simulink model "Repetitive_Controller"  (R2021b)
settings: Solver=FixedStepDiscrete  StartTime=0.0  StopTime=tspan(2)  FixedStep=0.1  RelTol=1e-3  EnableMultiTasking=on
undefined symbols (not defined in the file): K1, K2, Tmax, x_0
libraries: simulink x1
(part 1 of 2)
settings Model: Creator=domin  LastModifiedBy=domin
settings SolverCC: AlgebraicLoopSolver=TrustRegion  AutoInsertRateTranBlk=on
settings DataIOCC: LimitDataPoints=on
settings OptimizationCC: LifeSpan=inf
settings DebuggingCC: AllowSymbolicDim=off  SFUnexpectedBacktrackingDiag=warning  SFNoUnconditionalDefaultTransitionDiag=warning  SFExecutionAtInitializationDiag=none  ArithmeticOperatorsInVariantConditions=warning
settings SFSimCC: SimUseLocalCustomCode=off  CustomCodeUndefinedFunction=UseInterfaceOnly
settings RTWCC: RTWUseLocalCustomCode=off
settings CodeAppCC: StateflowObjectComments=on
settings GRTTargetCC: TargetLangStandard=C89/C90 (ANSI)
settings ConfigComp: CovMetricSettings=dw  CovSaveCumulativeToWorkspaceVar=on  CovSaveSingleToWorkspaceVar=on  CovExternalEMLEnable=off  CovSFcnEnable=off

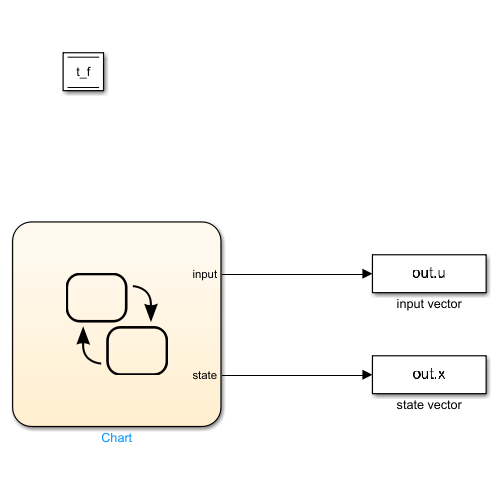
[thumbnail: Simulink's stored preview of the top-level diagram]
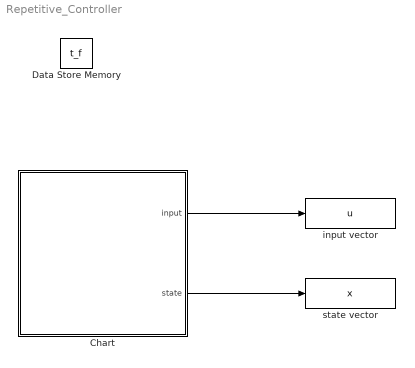
== system Repetitive_Controller ==
  Chart : Stateflow chart  TreatAsAtomicUnit=on
  Data Store Memory : DataStoreMemory  DataStoreName=t_f  ReadBeforeWriteMsg=warning  WriteAfterWriteMsg=warning  WriteAfterReadMsg=warning  ShowAdditionalParam=off
  input vector : ToWorkspace  VariableName=u  SampleTime=-1
  state vector : ToWorkspace  VariableName=x  SampleTime=-1
  wires:
  Chart/2(state) -> state vector/1
  Chart/1(input) -> input vector/1

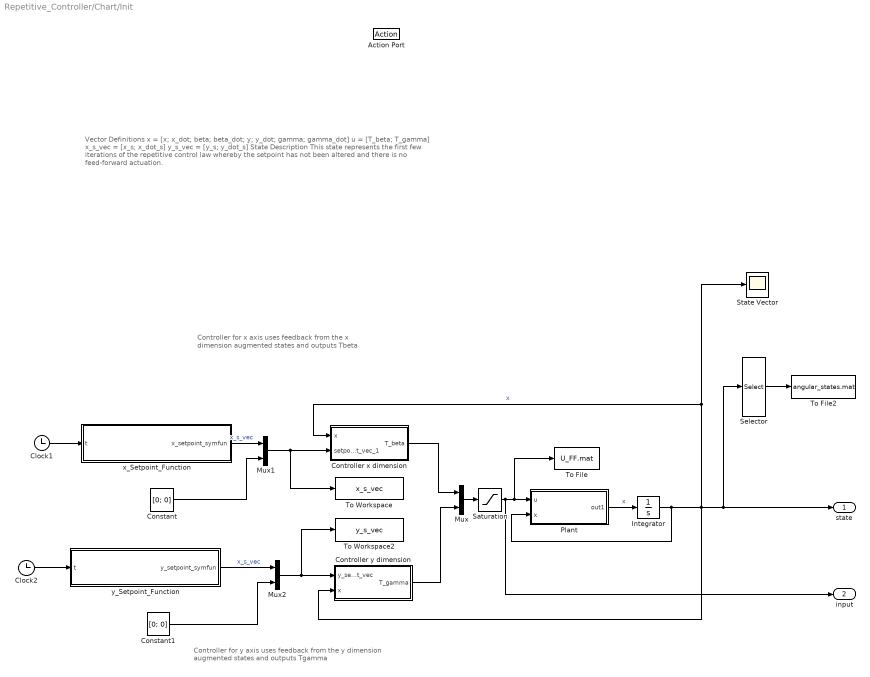
== system Repetitive_Controller/Chart/Init ==
  note: Controller for y axis uses feedback from the
      | y dimension augmented states and outputs Tgamma
  note: Vector Definitions
      |
      | x = [x; x_dot; beta; beta_dot; y; y_dot; gamma; gamma_dot]
      | u = [T_beta; T_gamma]
      | x_s_vec = [x_s; x_dot_s]
      | y_s_vec = [y_s; y_dot_s]
      |
      | State Description
      | This state represents the first few iterations of the repetitive control law whereby the setpoint has not been altered and there is no feed-forward actuation.
  note: Controller for x axis uses feedback from the
      | x dimension augmented states and outputs Tbeta
  Action Port : ActionPort
      settings: CopyFcn=Stateflow.SLINSF.SimulinkMan.removeBlockPreDeleteFcn  PreDeleteFcn=Stateflow.SLINSF.SimulinkMan.unsafePredeleteFcn
  Clock1 : Clock
  Clock2 : Clock
  Constant : Constant  Value=[0; 0]
  Constant1 : Constant  Value=[0; 0]
  Controller x dimension : Subsystem
  Controller y dimension : Subsystem
  Integrator : Integrator  InitialCondition=x_0  ContinuousStateAttributes='x'
  Mux : Mux  Inputs=2
  Mux1 : Mux  Inputs=2
  Mux2 : Mux  Inputs=2
  Plant : Subsystem
  Saturation : Saturate  UpperLimit=Tmax  LowerLimit=-Tmax
  Selector : Selector  InputPortWidth=8  IndexOptions=Index vector (dialog)  Indices=[3 4 7 8]  OutputSizes=1
  State Vector : Scope
  To File : ToFile  Filename=U_FF.mat
  To File2 : ToFile  Filename=angular_states.mat
  To Workspace : ToWorkspace  VariableName=x_s_vec  SampleTime=-1
  To Workspace2 : ToWorkspace  VariableName=y_s_vec  SampleTime=-1
  x_Setpoint_Function : MATLAB Function  TreatAsAtomicUnit=on
  y_Setpoint_Function : MATLAB Function  TreatAsAtomicUnit=on
  state : Outport
  input : Outport  Port=2
  wires:
  Saturation/1 -> input/1, To File/1, Plant/1(u)
  Clock2/1 -> y_Setpoint_Function/1(t)
  Mux/1 -> Saturation/1
  Clock1/1 -> x_Setpoint_Function/1(t)
  Plant/1(out1) -> Integrator/1  "x"
  Controller x dimension/1(T_beta) -> Mux/1
  x_Setpoint_Function/1(x_setpoint_symfun) -> Mux1/1  "x_s_vec"
  Controller y dimension/1(T_gamma) -> Mux/2
  Mux1/1 -> To Workspace/1, Controller x dimension/2(setpoint_vec_1)
  Constant/1 -> Mux1/2
  Mux2/1 -> To Workspace2/1, Controller y dimension/1(y_setpoint_vec)
  y_Setpoint_Function/1(y_setpoint_symfun) -> Mux2/1  "x_s_vec"
  Constant1/1 -> Mux2/2
  Selector/1 -> To File2/1
  Integrator/1 -> Plant/2(x), state/1, Selector/1, Controller x dimension/1(x), State Vector/1, Controller y dimension/2(x)  "x"

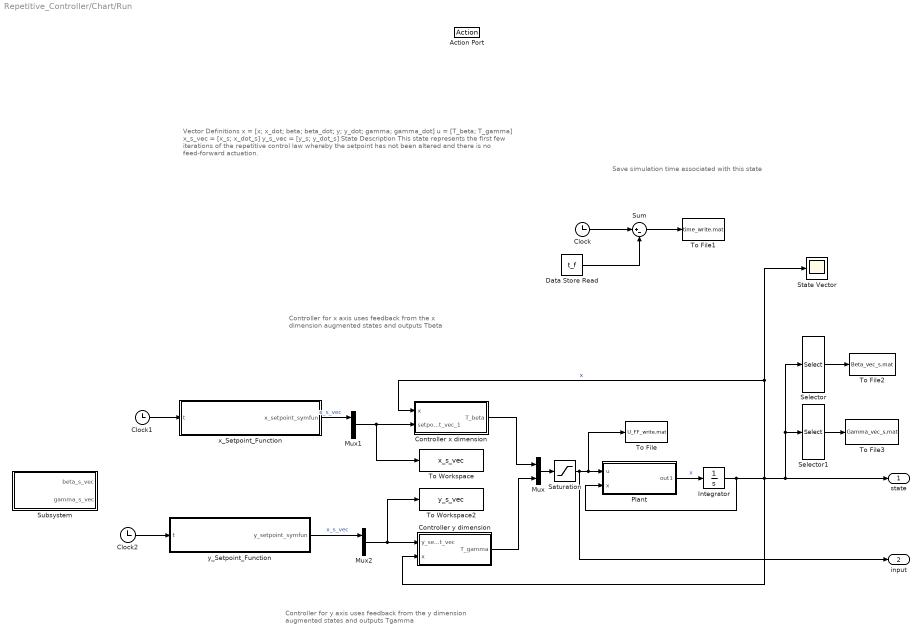
== system Repetitive_Controller/Chart/Run ==
  note: Save simulation time associated with this state
  note: Controller for y axis uses feedback from the
      | y dimension augmented states and outputs Tgamma
  note: Vector Definitions
      |
      | x = [x; x_dot; beta; beta_dot; y; y_dot; gamma; gamma_dot]
      | u = [T_beta; T_gamma]
      | x_s_vec = [x_s; x_dot_s]
      | y_s_vec = [y_s; y_dot_s]
      |
      | State Description
      | This state represents the first few iterations of the repetitive control law whereby the setpoint has not been altered and there is no feed-forward actuation.
  note: Controller for x axis uses feedback from the
      | x dimension augmented states and outputs Tbeta
  Action Port : ActionPort
      settings: CopyFcn=Stateflow.SLINSF.SimulinkMan.removeBlockPreDeleteFcn  PreDeleteFcn=Stateflow.SLINSF.SimulinkMan.unsafePredeleteFcn
  Clock : Clock
  Clock1 : Clock
  Clock2 : Clock
  Controller x dimension : Subsystem
  Controller y dimension : Subsystem
  Data Store Read : DataStoreRead  DataStoreName=t_f  IndexOptions=Index vector (dialog)  Indices=1  OutputSizes=1
  Integrator : Integrator  ContinuousStateAttributes='x'
  Mux : Mux  Inputs=2
  Mux1 : Mux  Inputs=2
  Mux2 : Mux  Inputs=2
  Plant : Subsystem
  Saturation : Saturate  UpperLimit=Tmax  LowerLimit=-Tmax
  Selector : Selector  InputPortWidth=8  IndexOptions=Index vector (dialog)  Indices=[3 4]  OutputSizes=1
  Selector1 : Selector  InputPortWidth=8  IndexOptions=Index vector (dialog)  Indices=[7 8]  OutputSizes=1
  State Vector : Scope
  Subsystem : Subsystem
  Sum : Sum  Inputs=|+-
  To File : ToFile  Filename=U_FF_write.mat
  To File1 : ToFile  Filename=time_write.mat
  To File2 : ToFile  Filename=Beta_vec_s.mat
  To File3 : ToFile  Filename=Gamma_vec_s.mat
  To Workspace : ToWorkspace  VariableName=x_s_vec  SampleTime=-1
  To Workspace2 : ToWorkspace  VariableName=y_s_vec  SampleTime=-1
  x_Setpoint_Function : MATLAB Function  TreatAsAtomicUnit=on
  y_Setpoint_Function : MATLAB Function  TreatAsAtomicUnit=on
  " state" : Outport
  input : Outport  Port=2
  wires:
  Saturation/1 -> input/1, To File/1, Plant/1(u)
  Clock2/1 -> y_Setpoint_Function/1(t)
  Mux/1 -> Saturation/1
  Clock1/1 -> x_Setpoint_Function/1(t)
  Plant/1(out1) -> Integrator/1  "x"
  Controller x dimension/1(T_beta) -> Mux/1
  x_Setpoint_Function/1(x_setpoint_symfun) -> Mux1/1  "x_s_vec"
  Controller y dimension/1(T_gamma) -> Mux/2
  Mux1/1 -> To Workspace/1, Controller x dimension/2(setpoint_vec_1)
  ? -> Mux1/2
  Mux2/1 -> To Workspace2/1, Controller y dimension/1(y_setpoint_vec)
  y_Setpoint_Function/1(y_setpoint_symfun) -> Mux2/1  "x_s_vec"
  ? -> Mux2/2
  Clock/1 -> Sum/1
  Sum/1 -> To File1/1
  Data Store Read/1 -> Sum/2
  Selector/1 -> To File2/1
  Selector1/1 -> To File3/1
  Integrator/1 -> Plant/2(x), " state"/1, Selector1/1, Selector/1, Controller x dimension/1(x), State Vector/1, Controller y dimension/2(x)  "x"

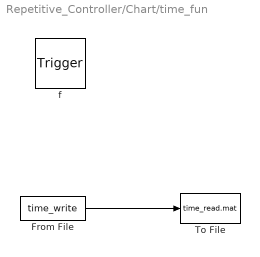
== system Repetitive_Controller/Chart/time_fun ==
  f : TriggerPort  TriggerType=function-call  VariantControl=(inherit)
      settings: CopyFcn=Stateflow.SLINSF.SimulinkMan.removeBlockPreDeleteFcn  PreDeleteFcn=Stateflow.SLINSF.SimulinkMan.unsafePredeleteFcn
  From File : FromFile  FileName=time_write  SampleTime=0
  To File : ToFile  Filename=time_read.mat  SaveFormat=Timeseries
  wires:
  From File/1 -> To File/1

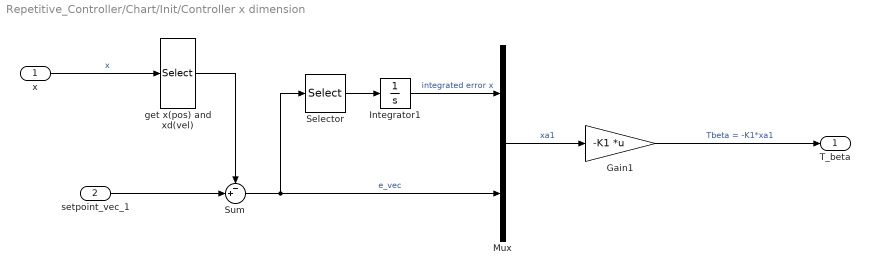
== system Repetitive_Controller/Chart/Init/Controller x dimension ==
  x : Inport
  setpoint_vec_1 : Inport  Port=2
  Gain1 : Gain  Gain=-K1  Multiplication=Matrix(K*u)
  Integrator1 : Integrator
  Mux : Mux  Inputs=2
  Selector : Selector  InputPortWidth=4  IndexOptions=Index vector (dialog)  Indices=[1 ]  OutputSizes=1
  Sum : Sum  Inputs=-+|
  get x(pos) and xd(vel) : Selector  InputPortWidth=8  IndexOptions=Index vector (dialog)  Indices=[1:4]  OutputSizes=1
  T_beta : Outport
  wires:
  Gain1/1 -> T_beta/1  "Tbeta = -K1*xa1"
  get x(pos) and xd(vel)/1 -> Sum/1
  Mux/1 -> Gain1/1  "xa1"
  Sum/1 -> Selector/1, Mux/2  "e_vec"
  setpoint_vec_1/1 -> Sum/2
  x/1 -> get x(pos) and xd(vel)/1  "x"
  Selector/1 -> Integrator1/1
  Integrator1/1 -> Mux/1  "integrated error x"

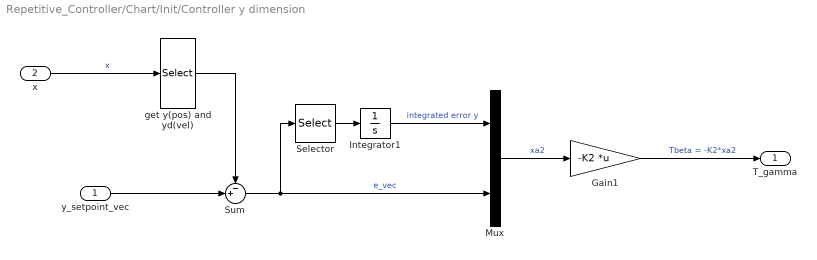
== system Repetitive_Controller/Chart/Init/Controller y dimension ==
  y_setpoint_vec : Inport
  x : Inport  Port=2
  Gain1 : Gain  Gain=-K2  Multiplication=Matrix(K*u)
  Integrator1 : Integrator
  Mux : Mux  Inputs=2
  Selector : Selector  InputPortWidth=4  IndexOptions=Index vector (dialog)  Indices=[1 ]  OutputSizes=1
  Sum : Sum  Inputs=-+|
  get y(pos) and yd(vel) : Selector  InputPortWidth=8  IndexOptions=Index vector (dialog)  Indices=[5:8]  OutputSizes=1
  T_gamma : Outport
  wires:
  Integrator1/1 -> Mux/1  "integrated error y"
  x/1 -> get y(pos) and yd(vel)/1  "x"
  Gain1/1 -> T_gamma/1  "Tbeta = -K2*xa2"
  get y(pos) and yd(vel)/1 -> Sum/1
  Mux/1 -> Gain1/1  "xa2"
  Selector/1 -> Integrator1/1
  Sum/1 -> Selector/1, Mux/2  "e_vec"
  y_setpoint_vec/1 -> Sum/2

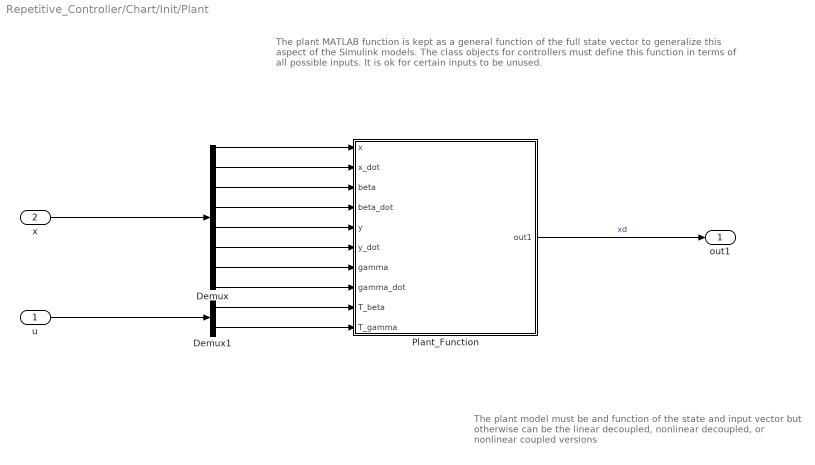
== system Repetitive_Controller/Chart/Init/Plant ==
  note: The plant MATLAB function is kept as a general function of the full state vector
      | to generalize this aspect of the Simulink models. The class objects for controllers must define this function in terms of all possible inputs. It is ok for certain inputs to be unused.
  note: The plant model must be and function of the state and input vector
      |  but otherwise can be the linear decoupled, nonlinear decoupled,
      | or nonlinear coupled versions
  u : Inport
  x : Inport  Port=2
  Demux : Demux  Outputs=8
  Demux1 : Demux  Outputs=2
  Plant_Function : MATLAB Function  TreatAsAtomicUnit=on
  out1 : Outport
  wires:
  Demux1/1 -> Plant_Function/9(T_beta)
  Demux1/2 -> Plant_Function/10(T_gamma)
  Demux/5 -> Plant_Function/5(y)
  Demux/8 -> Plant_Function/8(gamma_dot)
  Demux/7 -> Plant_Function/7(gamma)
  Demux/1 -> Plant_Function/1(x)
  Demux/3 -> Plant_Function/3(beta)
  Demux/4 -> Plant_Function/4(beta_dot)
  Demux/2 -> Plant_Function/2(x_dot)
  Demux/6 -> Plant_Function/6(y_dot)
  x/1 -> Demux/1
  Plant_Function/1(out1) -> out1/1  "xd"
  u/1 -> Demux1/1

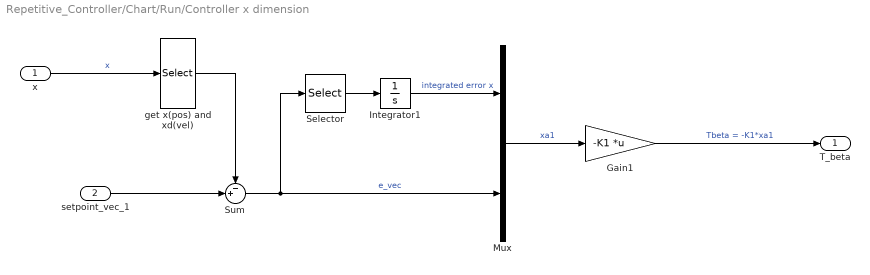
== system Repetitive_Controller/Chart/Run/Controller x dimension ==
  x : Inport
  setpoint_vec_1 : Inport  Port=2
  Gain1 : Gain  Gain=-K1  Multiplication=Matrix(K*u)
  Integrator1 : Integrator
  Mux : Mux  Inputs=2
  Selector : Selector  InputPortWidth=4  IndexOptions=Index vector (dialog)  Indices=[1 ]  OutputSizes=1
  Sum : Sum  Inputs=-+|
  get x(pos) and xd(vel) : Selector  InputPortWidth=8  IndexOptions=Index vector (dialog)  Indices=[1:4]  OutputSizes=1
  T_beta : Outport
  wires:
  Gain1/1 -> T_beta/1  "Tbeta = -K1*xa1"
  get x(pos) and xd(vel)/1 -> Sum/1
  Mux/1 -> Gain1/1  "xa1"
  Sum/1 -> Selector/1, Mux/2  "e_vec"
  setpoint_vec_1/1 -> Sum/2
  x/1 -> get x(pos) and xd(vel)/1  "x"
  Selector/1 -> Integrator1/1
  Integrator1/1 -> Mux/1  "integrated error x"

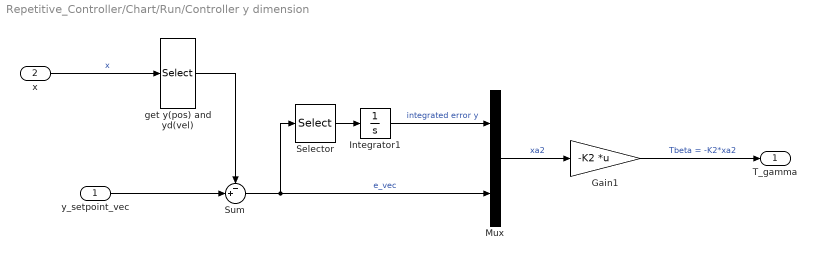
== system Repetitive_Controller/Chart/Run/Controller y dimension ==
  y_setpoint_vec : Inport
  x : Inport  Port=2
  Gain1 : Gain  Gain=-K2  Multiplication=Matrix(K*u)
  Integrator1 : Integrator
  Mux : Mux  Inputs=2
  Selector : Selector  InputPortWidth=4  IndexOptions=Index vector (dialog)  Indices=[1 ]  OutputSizes=1
  Sum : Sum  Inputs=-+|
  get y(pos) and yd(vel) : Selector  InputPortWidth=8  IndexOptions=Index vector (dialog)  Indices=[5:8]  OutputSizes=1
  T_gamma : Outport
  wires:
  Integrator1/1 -> Mux/1  "integrated error y"
  x/1 -> get y(pos) and yd(vel)/1  "x"
  Gain1/1 -> T_gamma/1  "Tbeta = -K2*xa2"
  get y(pos) and yd(vel)/1 -> Sum/1
  Mux/1 -> Gain1/1  "xa2"
  Selector/1 -> Integrator1/1
  Sum/1 -> Selector/1, Mux/2  "e_vec"
  y_setpoint_vec/1 -> Sum/2

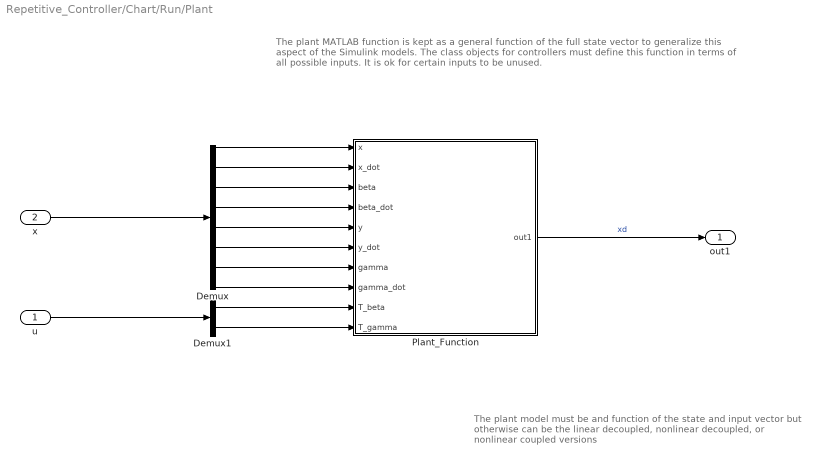
== system Repetitive_Controller/Chart/Run/Plant ==
  note: The plant MATLAB function is kept as a general function of the full state vector
      | to generalize this aspect of the Simulink models. The class objects for controllers must define this function in terms of all possible inputs. It is ok for certain inputs to be unused.
  note: The plant model must be and function of the state and input vector
      |  but otherwise can be the linear decoupled, nonlinear decoupled,
      | or nonlinear coupled versions
  u : Inport
  x : Inport  Port=2
  Demux : Demux  Outputs=8
  Demux1 : Demux  Outputs=2
  Plant_Function : MATLAB Function  TreatAsAtomicUnit=on
  out1 : Outport
  wires:
  Demux1/1 -> Plant_Function/9(T_beta)
  Demux1/2 -> Plant_Function/10(T_gamma)
  Demux/5 -> Plant_Function/5(y)
  Demux/8 -> Plant_Function/8(gamma_dot)
  Demux/7 -> Plant_Function/7(gamma)
  Demux/1 -> Plant_Function/1(x)
  Demux/3 -> Plant_Function/3(beta)
  Demux/4 -> Plant_Function/4(beta_dot)
  Demux/2 -> Plant_Function/2(x_dot)
  Demux/6 -> Plant_Function/6(y_dot)
  x/1 -> Demux/1
  Plant_Function/1(out1) -> out1/1  "xd"
  u/1 -> Demux1/1

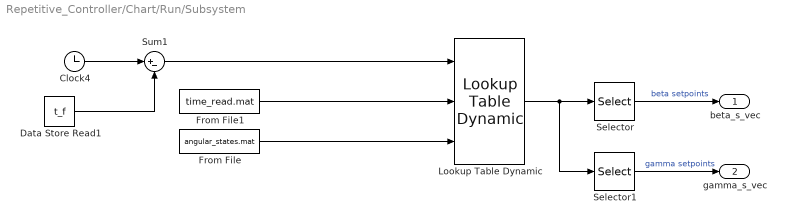
== system Repetitive_Controller/Chart/Run/Subsystem ==
  Clock4 : Clock
  Data Store Read1 : DataStoreRead  DataStoreName=t_f  IndexOptions=Index vector (dialog)  Indices=1  OutputSizes=1
  From File : FromFile  FileName=angular_states.mat  SampleTime=0
  From File1 : FromFile  FileName=time_read.mat  SampleTime=0
  Lookup Table Dynamic : simulink/Lookup Tables/Lookup Table Dynamic  LookUpMeth=Interpolation-Extrapolation  OutDataType=fixdt('double')  OutScaling=2^-10  OutputDataTypeScalingMode=Specify via dialog  OutDataTypeStr=double  DoSatur=off
  Selector : Selector  InputPortWidth=4  IndexOptions=Index vector (dialog)  Indices=[1 2]  OutputSizes=1
  Selector1 : Selector  InputPortWidth=4  IndexOptions=Index vector (dialog)  Indices=[3 4]  OutputSizes=1
  Sum1 : Sum  Inputs=|+-
  beta_s_vec : Outport
  gamma_s_vec : Outport  Port=2
  wires:
  Data Store Read1/1 -> Sum1/2
  From File/1 -> Lookup Table Dynamic/3
  Lookup Table Dynamic/1 -> Selector1/1, Selector/1
  Sum1/1 -> Lookup Table Dynamic/1
  From File1/1 -> Lookup Table Dynamic/2
  Clock4/1 -> Sum1/1
  Selector/1 -> beta_s_vec/1  "beta setpoints"
  Selector1/1 -> gamma_s_vec/1  "gamma setpoints"

== matlab function Repetitive_Controller/Chart/Init/Plant/Plant_Function ==
  data: x input; out1 output size=8; x_dot input; beta input; beta_dot input; y input; y_dot input; gamma input; gamma_dot input; T_beta input; T_gamma input
function out1 = xdot(x,x_dot,beta,beta_dot,y,y_dot,gamma,gamma_dot,T_beta,T_gamma)
%#codegen

%    This function was generated by the Symbolic Math Toolbox version 9.0.
%    10-Dec-2021 15:41:41

t2 = cos(beta);
t3 = cos(gamma);
t4 = sin(beta);
t5 = sin(gamma);
t6 = beta_dot.^2;
t7 = gamma_dot.^2;
t8 = x.^2;
t9 = x.^3;
t10 = y.^2;
t11 = y.^3;
t13 = y.^5;
t12 = t10.^2;
t14 = t3.^2;
t15 = t3.^3;
t17 = t3.^5;
t19 = t5.^2;
t20 = t5.^3;
t22 = t5.^5;
t29 = t3.*t5.*t8.*y.*1.35016875e-1;
t36 = t3.*t5.*y.*2.54260666546875e-1;
t16 = t14.^2;
t18 = t14.^3;
t21 = t19.^2;
t24 = t8.*t19.*1.24425;
t26 = t12.*t14.*t19.*(5.67e+2./1.6e+2);
t27 = t3.*t11.*t20.*7.2646875e-1;
t28 = t5.*t11.*t15.*7.2646875e-1;
t30 = t8.*t10.*t14.*t19.*(5.67e+2./1.6e+2);
t31 = -t29;
t32 = t3.*t8.*t20.*y.*8.61485625e-1;
t33 = t5.*t8.*t15.*y.*8.61485625e-1;
t34 = t10.*t19.*1.240295934375;
t35 = t8.*t14.*4.3410357703125;
t39 = t19.*2.520596373817331e-3;
t42 = t3.*t20.*y.*9.746092345495838e-2;
t43 = t5.*t15.*y.*9.746092345495838e-2;
t44 = t8.*t14.*t19.*2.124794480871038;
t45 = t10.*t14.*t19.*6.487623695046038;
t46 = t14.*2.101722893640155;
t49 = t14.*t19.*8.065797848171603e-1;
t23 = t12.*t21.*(5.67e+2./1.6e+2);
t25 = t8.*t10.*t21.*(5.67e+2./1.6e+2);
t37 = t10.*t21.*4.82620938917175e-1;
t38 = t8.*t21.*4.60827495054675e-1;
t40 = t8.*t16.*1.663966985816362;
t41 = t10.*t16.*6.005002756128863;
t47 = t21.*9.66172446512356e-4;
t48 = t16.*8.056136123706479e-1;
t50 = t23+t24+t25+t26+t27+t28+t30+t31+t32+t33+t34+t35+t36+t37+t38+t39+t40+t41+t42+t43+t44+t45+t46+t47+t48+t49;
t51 = 1.0./t50;
et1 = T_beta.*t3.*(-2.1476413157)-T_beta.*t15.*8.232146510146728e-1+t4.*t14.*7.39780227196038+t4.*t16.*2.835659367822534;
et2 = t4.*t19.*1.76621788765343e-2+t4.*t21.*6.770108357347294e-3-T_beta.*t3.*t19.*8.232146510146728e-1-T_beta.*t10.*t15.*6.1362-T_beta.*t11.*t20.*(3.15e+2./8.0)+beta_dot.*gamma_dot.*t20.*5.337182778960069e-4;
et3 = beta_dot.*gamma_dot.*t22.*2.045801143172306e-4-T_beta.*t5.*y.*1.37810659375e+1-T_beta.*t20.*y.*5.2824348756075-beta_dot.*t20.*y_dot.*4.321022355115425e-3-beta_dot.*t22.*y_dot.*1.65629562259261e-3;
et4 = t4.*t8.*t14.*3.041825779054688e+1+t4.*t8.*t16.*1.165965437918465e+1+t6.*t9.*t14.*3.1007398359375+t4.*t10.*t16.*2.113686022398367e+1+t4.*t8.*t19.*8.7186375+t6.*t9.*t16.*1.188547847011688;
et5 = t4.*t8.*t21.*3.229084090347401+t6.*t9.*t19.*(7.11e+2./8.0e+2)+t4.*t10.*t21.*5.0464042216875e-2+t6.*t9.*t21.*3.29162496467625e-1+t4.*t14.*t19.*2.842429476179882;
et6 = t2.*t3.*x.*(-4.740381294078825)-t2.*t15.*x.*1.817040538452137+t6.*t14.*x.*1.487079216073444+t7.*t14.*x.*6.79406330221695e-2;
et7 = t6.*t16.*x.*6.379545310329106e-1+t7.*t16.*x.*2.604239548484917e-2+t6.*t18.*x.*2.604239548484917e-2+t6.*t19.*x.*1.800425981298094e-3;
et8 = t6.*t21.*x.*6.901231760802543e-4-T_beta.*t5.*t11.*t14.*(3.15e+2./8.0)-T_beta.*t3.*t10.*t19.*6.1362-beta_dot.*gamma_dot.*t5.*t14.*2.313734573036617e-2-beta_dot.*gamma_dot.*t5.*t16.*8.868800321352103e-3;
et9 = beta_dot.*gamma_dot.*t8.*t20.*2.6346105e-1-beta_dot.*gamma_dot.*t11.*t17.*8.497709015898375+beta_dot.*gamma_dot.*t8.*t22.*9.757693045286275e-2+beta_dot.*gamma_dot.*t10.*t20.*4.72552750996875e-2+beta_dot.*gamma_dot.*t10.*t22.*1.963839892085062e-2+beta_dot.*gamma_dot.*t12.*t22.*1.35016875e-1;
et10 = beta_dot.*gamma_dot.*t14.*t20.*(-8.664220207034872e-3)+T_gamma.*t3.*t5.*x.*1.79703e-1-T_beta.*t5.*t14.*y.*5.2824348756075-beta_dot.*gamma_dot.*t15.*y.*2.974158432146889;
et11 = beta_dot.*gamma_dot.*t17.*y.*(-1.140027796021482)-T_gamma.*t14.*x.*y.*6.1362+T_gamma.*t19.*x.*y.*(3.69e+2./3.2e+2)-beta_dot.*t5.*t14.*y_dot.*3.596166371785134-beta_dot.*t5.*t16.*y_dot.*1.378450313419718;
et12 = beta_dot.*t8.*t20.*y_dot.*(-2.133)-beta_dot.*t8.*t22.*y_dot.*7.899899915223e-1-beta_dot.*t10.*t20.*y_dot.*1.240295934375-beta_dot.*t10.*t22.*y_dot.*4.87765081854675e-1-beta_dot.*t12.*t22.*y_dot.*(5.67e+2./1.6e+2)-beta_dot.*t14.*t20.*y_dot.*1.380106609042311;
et13 = beta_dot.*t15.*x.*x_dot.*9.66438592065e-1+beta_dot.*t17.*x.*x_dot.*3.704465929566028e-1-gamma_dot.*t3.*t5.*x_dot.*7.3642620715353e-3-gamma_dot.*t5.*t15.*x_dot.*2.822803038329313e-3;
et14 = gamma_dot.*t3.*t20.*x_dot.*(-2.822803038329313e-3)-gamma_dot.*t11.*t21.*x_dot.*1.35016875e-1-gamma_dot.*t14.*x.*y_dot.*9.66438592065e-1-gamma_dot.*t16.*x.*y_dot.*3.704465929566028e-1-gamma_dot.*t19.*x_dot.*y.*4.72552750996875e-2;
et15 = gamma_dot.*t21.*x_dot.*y.*(-1.811346918845812e-2)-t4.*t5.*t11.*t15.*1.331546137149375e+2-t3.*t4.*t11.*t20.*1.331546137149375e+2+t4.*t8.*t10.*t21.*2.48315625e+1+t4.*t8.*t14.*t19.*1.488873846953206e+1+t6.*t9.*t10.*t21.*(8.1e+1./3.2e+1);
et16 = t4.*t10.*t14.*t19.*2.118732426620054e+1+t6.*t9.*t14.*t19.*1.517710343479313+t2.*t3.*t19.*x.*2.222054701596104+t2.*t3.*t21.*x.*1.258051161599348-t6.*t10.*t14.*x.*1.5029307e-2;
et17 = t7.*t10.*t14.*x.*(-1.5029307e-2)+t6.*t10.*t16.*x.*4.319346296949187-t2.*t11.*t20.*x.*8.691046875e+1+t7.*t10.*t16.*x.*5.5462482e-2-t6.*t10.*t18.*x.*5.5462482e-2+t2.*t11.*t22.*x.*6.207890625e+1+t6.*t10.*t19.*x.*(7.11e+2./8.0e+2)+t2.*t15.*t19.*x.*1.258051161599348;
et18 = t7.*t10.*t19.*x.*(7.11e+2./8.0e+2)+t6.*t10.*t21.*x.*3.34306639405125e-1+t7.*t10.*t21.*x.*3.65641605842625e-1+t6.*t12.*t21.*x.*(8.1e+1./3.2e+1)+t6.*t14.*t19.*x.*5.759809778668214e-1+t7.*t12.*t21.*x.*(8.1e+1./3.2e+1);
et19 = t7.*t14.*t19.*x.*2.604239548484917e-2+t6.*t14.*t21.*x.*1.954403639426509e-3+t6.*t16.*t19.*x.*2.799679912427568e-2-t3.*t4.*t5.*y.*4.660349235524814e+1;
et20 = t4.*t5.*t15.*y.*(-1.786363365932268e+1)-t3.*t4.*t20.*y.*1.786363365932268e+1-t2.*t5.*x.*y.*3.041825779054688e+1+t2.*t20.*x.*y.*1.425856456363003e+1;
et21 = t2.*t22.*x.*y.*8.072710225868503+beta_dot.*gamma_dot.*t5.*t8.*t14.*9.191833169653125e-1+beta_dot.*gamma_dot.*t5.*t8.*t16.*3.523331237681446e-1+beta_dot.*gamma_dot.*t5.*t10.*t14.*9.4510550199375e-2-beta_dot.*gamma_dot.*t5.*t10.*t16.*2.988064664334938e-2;
et22 = beta_dot.*gamma_dot.*t5.*t12.*t16.*2.7003375e-1-beta_dot.*gamma_dot.*t3.*t11.*t21.*8.535675761148375+beta_dot.*gamma_dot.*t8.*t10.*t22.*7.5036375e-1+beta_dot.*gamma_dot.*t8.*t14.*t20.*4.499100542210074e-1-beta_dot.*gamma_dot.*t10.*t14.*t20.*1.024224772249876e-2-beta_dot.*gamma_dot.*t11.*t15.*t19.*1.703338477704675e+1;
et23 = beta_dot.*gamma_dot.*t12.*t14.*t20.*4.05050625e-1-T_gamma.*t3.*t5.*t10.*x.*(3.15e+2./8.0)-beta_dot.*gamma_dot.*t3.*t19.*y.*2.987446615504921-beta_dot.*gamma_dot.*t8.*t15.*y.*6.201479671875-beta_dot.*gamma_dot.*t3.*t21.*y.*1.145121303557277-beta_dot.*gamma_dot.*t8.*t17.*y.*2.377095694023375;
et24 = beta_dot.*gamma_dot.*t15.*t19.*y.*(-2.285149099578759)-beta_dot.*t5.*t8.*t14.*y_dot.*7.44177560625-beta_dot.*t5.*t8.*t16.*y_dot.*2.85251483282805-beta_dot.*t5.*t10.*t16.*y_dot.*1.027489829387805e+1-beta_dot.*t3.*t11.*t21.*y_dot.*7.2646875e-1-beta_dot.*t8.*t10.*t22.*y_dot.*(2.43e+2./4.0e+1);
et25 = beta_dot.*t8.*t14.*t20.*y_dot.*(-3.64250482435035)-beta_dot.*t10.*t14.*t20.*y_dot.*1.076266337573272e+1-beta_dot.*t11.*t15.*t19.*y_dot.*7.2646875e-1-beta_dot.*t12.*t14.*t20.*y_dot.*(5.67e+2./1.6e+2)+beta_dot.*t3.*t19.*x.*x_dot.*1.385028e-1+beta_dot.*t3.*t21.*x.*x_dot.*5.129668344951468e-2+beta_dot.*t11.*t22.*x.*x_dot.*(8.1e+1./3.2e+1);
et26 = beta_dot.*t15.*t19.*x.*x_dot.*4.217432764061174e-1-gamma_dot.*t5.*t10.*t15.*x_dot.*2.10410298e-2-gamma_dot.*t3.*t10.*t20.*x_dot.*2.10410298e-2-gamma_dot.*t11.*t14.*t19.*x_dot.*1.35016875e-1-beta_dot.*t3.*t19.*y.*y_dot.*2.54260666546875e-1-beta_dot.*t3.*t21.*y.*y_dot.*9.746092345495838e-2;
et27 = beta_dot.*t15.*t19.*y.*y_dot.*(-9.746092345495838e-2)+beta_dot.*t20.*x.*x_dot.*y.*(7.11e+2./8.0e+2)+beta_dot.*t22.*x.*x_dot.*y.*3.29162496467625e-1-gamma_dot.*t10.*t21.*x.*y_dot.*5.1890625e-1-gamma_dot.*t14.*t19.*x.*y_dot.*3.704465929566028e-1-gamma_dot.*t14.*t19.*x_dot.*y.*1.811346918845812e-2;
et28 = t4.*t8.*t10.*t14.*t19.*2.48315625e+1+t6.*t9.*t10.*t14.*t19.*(8.1e+1./3.2e+1)-t3.*t5.*t6.*t11.*x.*9.6440625e-2-t3.*t5.*t7.*t11.*x.*9.6440625e-2-t2.*t3.*t10.*t19.*x.*1.591929901524375e+2+t2.*t3.*t10.*t21.*x.*1.840267096875e+1+t5.*t6.*t11.*t15.*x.*7.117875e-1+t5.*t7.*t11.*t15.*x.*7.5036375e-1-t5.*t6.*t11.*t17.*x.*7.5036375e-1;
et29 = t3.*t6.*t11.*t20.*x.*6.15346875e-1+t3.*t7.*t11.*t20.*x.*7.5036375e-1+t3.*t6.*t11.*t22.*x.*6.15346875e-1+t2.*t10.*t15.*t19.*x.*1.840267096875e+1+t2.*t11.*t14.*t20.*x.*6.207890625e+1+t6.*t10.*t14.*t19.*x.*9.947678913416812+t7.*t10.*t14.*t19.*x.*4.21104087842625e-1;
et30 = t6.*t10.*t14.*t21.*x.*2.19386751580575+t6.*t10.*t16.*t19.*x.*2.13840503380575+t6.*t12.*t14.*t19.*x.*(8.1e+1./3.2e+1)-t6.*t11.*t15.*t20.*x.*1.35016875e-1+t7.*t12.*t14.*t19.*x.*(8.1e+1./3.2e+1)-t6.*t12.*t14.*t21.*x.*(8.1e+1./3.2e+1)-t6.*t12.*t16.*t19.*x.*(8.1e+1./3.2e+1)-t3.*t4.*t5.*t8.*y.*9.4608253125e-1-t3.*t5.*t6.*t9.*y.*9.6440625e-2;
et31 = t4.*t5.*t8.*t15.*y.*6.03655284375+t3.*t4.*t8.*t20.*y.*6.03655284375+t5.*t6.*t9.*t15.*y.*6.15346875e-1+t3.*t6.*t9.*t20.*y.*6.15346875e-1+t3.*t5.*t6.*x.*y.*9.12475249003125e-2+t3.*t5.*t7.*x.*y.*5.744668209328125e-1-t2.*t5.*t14.*x.*y.*3.435757314273251e+1;
et32 = t2.*t5.*t16.*x.*y.*1.36021737105+t5.*t6.*t15.*x.*y.*1.296510410662169+t5.*t7.*t15.*x.*y.*2.240914151443579e-1+t5.*t6.*t17.*x.*y.*4.940577617661313e-1+t3.*t6.*t20.*x.*y.*6.704458926105656e-2;
et33 = t3.*t7.*t20.*x.*y.*2.240914151443579e-1+t3.*t6.*t22.*x.*y.*1.254109111541651e-2+t2.*t14.*t20.*x.*y.*9.432927596918503+t6.*t15.*t20.*x.*y.*5.065988528815479e-1-beta_dot.*t8.*t10.*t14.*t20.*y_dot.*(2.43e+2./4.0e+1)-beta_dot.*t3.*t10.*t19.*x.*x_dot.*9.6440625e-2;
et34 = beta_dot.*t3.*t10.*t21.*x.*x_dot.*1.26927+beta_dot.*t10.*t15.*t19.*x.*x_dot.*1.26927+beta_dot.*t11.*t14.*t20.*x.*x_dot.*(8.1e+1./3.2e+1)+beta_dot.*t3.*t8.*t19.*y.*y_dot.*2.314575e-1-beta_dot.*t3.*t8.*t21.*y.*y_dot.*1.4768325-beta_dot.*t8.*t15.*t19.*y.*y_dot.*1.4768325+beta_dot.*t5.*t14.*x.*x_dot.*y.*6.186450364875+beta_dot.*t5.*t16.*x.*x_dot.*y.*2.513424526023375;
et35 = beta_dot.*t14.*t20.*x.*x_dot.*y.*2.842587022491-gamma_dot.*t10.*t14.*t19.*x.*y_dot.*5.1890625e-1-gamma_dot.*t3.*t5.*x.*y.*y_dot.*6.201479671875-gamma_dot.*t5.*t15.*x.*y.*y_dot.*2.457962044023375-gamma_dot.*t3.*t20.*x.*y.*y_dot.*2.457962044023375+beta_dot.*gamma_dot.*t5.*t8.*t10.*t14.*1.9288125e-1-beta_dot.*gamma_dot.*t5.*t8.*t10.*t16.*1.23069375;
et36 = beta_dot.*gamma_dot.*t3.*t8.*t11.*t21.*(-8.1e+1./1.6e+1)-beta_dot.*gamma_dot.*t8.*t10.*t14.*t20.*4.8033e-1-beta_dot.*gamma_dot.*t8.*t11.*t15.*t19.*(8.1e+1./1.6e+1)-beta_dot.*gamma_dot.*t3.*t8.*t19.*y.*1.806088858875-beta_dot.*gamma_dot.*t3.*t8.*t21.*y.*4.7591156531025e-1-beta_dot.*gamma_dot.*t8.*t15.*t19.*y.*2.853007259333625;
et37 = T_beta.*(-1.92934923125e+1)-T_beta.*t14.*7.3954088258505-T_beta.*t19.*7.3954088258505-t3.*t4.*6.584303391854071e+1-t4.*t15.*2.523836256676404e+1;
et38 = t2.*x.*(-4.258556090676563e+1)-T_beta.*t10.*t14.*(4.41e+2./8.0)-T_beta.*t10.*t19.*(4.41e+2./8.0)+T_gamma.*t5.*x.*1.614375-gamma_dot.*t5.*x_dot.*6.61573851395625e-2-gamma_dot.*t20.*x_dot.*2.535885686384136e-2-t3.*t4.*t19.*2.523836256676404e+1;
et39 = t4.*t10.*t15.*(-1.881254666584125e+2)-t4.*t11.*t20.*3.47641875e+1-t3.*t6.*x.*1.271303332734375e-1+t3.*t7.*x.*6.103496293059375e-1-t2.*t14.*x.*1.632351613085852e+1+t2.*t19.*x.*1.996199038908205e+1;
et40 = t6.*t15.*x.*5.616191675784583e-1+t7.*t15.*x.*2.339537582057806e-1+t2.*t21.*x.*1.13017943162159e+1+t6.*t17.*x.*2.339537582057806e-1-t4.*t5.*y.*1.216730311621875e+1;
et41 = t4.*t20.*y.*(-4.663861751673862)-beta_dot.*gamma_dot.*t3.*t5.*4.20576885660421-beta_dot.*gamma_dot.*t5.*t15.*1.6121176828866;
et42 = beta_dot.*gamma_dot.*t3.*t20.*(-1.6121176828866)+beta_dot.*gamma_dot.*t11.*t16.*7.2646875e-1-beta_dot.*gamma_dot.*t11.*t21.*8.61485625e-1+beta_dot.*gamma_dot.*t14.*y.*2.54260666546875e-1+beta_dot.*gamma_dot.*t16.*y.*9.746092345495838e-2-beta_dot.*gamma_dot.*t19.*y.*3.015159416465625e-1;
et43 = beta_dot.*gamma_dot.*t21.*y.*(-1.155743926434165e-1)-T_gamma.*t3.*x.*y.*(4.41e+2./8.0)+beta_dot.*t3.*t5.*y_dot.*6.0972948133875e-2+beta_dot.*t5.*t15.*y_dot.*2.337160486363782e-2+beta_dot.*t3.*t20.*y_dot.*2.337160486363782e-2+beta_dot.*t11.*t21.*y_dot.*(5.67e+2./1.6e+2);
et44 = beta_dot.*t14.*x.*x_dot.*8.682071540625+beta_dot.*t16.*x.*x_dot.*3.327933971632725+beta_dot.*t19.*x.*x_dot.*1.24425+beta_dot.*t21.*x.*x_dot.*4.60827495054675e-1-gamma_dot.*t5.*t14.*x_dot.*2.535885686384136e-2-gamma_dot.*t10.*t20.*x_dot.*1.89023625e-1+beta_dot.*t19.*y.*y_dot.*1.240295934375;
et45 = beta_dot.*t21.*y.*y_dot.*4.75419138804675e-1-gamma_dot.*t3.*x.*y_dot.*8.682071540625-gamma_dot.*t15.*x.*y_dot.*3.327933971632725-t4.*t5.*t11.*t14.*3.47641875e+1-t3.*t4.*t10.*t19.*1.881254666584125e+2-t3.*t6.*t10.*x.*1.35016875e-1-t3.*t7.*t10.*x.*1.35016875e-1;
et46 = t3.*t6.*t19.*x.*(-1.324536727479187e-3)+t3.*t7.*t19.*x.*2.339537582057806e-1+t3.*t6.*t21.*x.*1.755752756158312e-2-t2.*t10.*t19.*x.*1.2167465625e+2+t6.*t10.*t15.*x.*2.7003375e-1+t7.*t10.*t15.*x.*4.9825125e-1+t2.*t10.*t21.*x.*8.691046875e+1;
et47 = t6.*t10.*t17.*x.*(-4.9825125e-1)+t2.*t14.*t19.*x.*1.13017943162159e+1+t7.*t11.*t20.*x.*(5.67e+2./1.6e+2)+t6.*t15.*t19.*x.*2.515112857673637e-1-t4.*t5.*t14.*y.*4.663861751673862+t5.*t6.*x.*y.*3.954065625e-3+t5.*t7.*x.*y.*1.24425;
et48 = t6.*t20.*x.*y.*(-1.459164375e-2)+t7.*t20.*x.*y.*5.11898248179675e-1+beta_dot.*gamma_dot.*t3.*t5.*t10.*2.48059186875-beta_dot.*gamma_dot.*t5.*t10.*t15.*1.106580466422338e+1+beta_dot.*gamma_dot.*t5.*t12.*t15.*(5.67e+2./8.0e+1)-beta_dot.*gamma_dot.*t3.*t10.*t20.*1.106580466422338e+1+beta_dot.*gamma_dot.*t3.*t12.*t20.*(5.67e+2./8.0e+1);
et49 = beta_dot.*gamma_dot.*t11.*t14.*t19.*(-1.35016875e-1)-beta_dot.*gamma_dot.*t14.*t19.*y.*1.811346918845812e-2+beta_dot.*t5.*t10.*t15.*y_dot.*1.7421075e-1+beta_dot.*t3.*t10.*t20.*y_dot.*1.7421075e-1+beta_dot.*t11.*t14.*t19.*y_dot.*(5.67e+2./1.6e+2)+beta_dot.*t10.*t21.*x.*x_dot.*(5.67e+2./1.6e+2)+beta_dot.*t14.*t19.*x.*x_dot.*3.7887614666874-gamma_dot.*t5.*t10.*t14.*x_dot.*1.89023625e-1;
et50 = beta_dot.*t14.*t19.*y.*y_dot.*4.75419138804675e-1-gamma_dot.*t3.*t19.*x.*y_dot.*3.327933971632725-gamma_dot.*t20.*x.*y.*y_dot.*7.2646875e-1+t5.*t7.*t11.*t14.*x.*(5.67e+2./1.6e+2)+t3.*t6.*t10.*t19.*x.*1.35016875e-1-t5.*t6.*t11.*t16.*x.*(5.67e+2./1.6e+2)+t3.*t7.*t10.*t19.*x.*4.9825125e-1+t3.*t6.*t10.*t21.*x.*8.61485625e-1+t2.*t10.*t14.*t19.*x.*8.691046875e+1;
et51 = t6.*t10.*t15.*t19.*x.*3.63234375e-1-t6.*t11.*t14.*t20.*x.*(5.67e+2./1.6e+2)-t2.*t3.*t5.*x.*y.*2.039084077834125e+2+t2.*t5.*t15.*x.*y.*1.221961190625e+1+t2.*t3.*t20.*x.*y.*1.221961190625e+1+t5.*t6.*t14.*x.*y.*7.4180857539375+t5.*t7.*t14.*x.*y.*5.11898248179675e-1;
et52 = t5.*t6.*t16.*x.*y.*2.93716060232805+t6.*t14.*t20.*x.*y.*2.93716060232805+beta_dot.*t10.*t14.*t19.*x.*x_dot.*(5.67e+2./1.6e+2)-beta_dot.*t3.*t5.*x.*x_dot.*y.*1.35016875e-1+beta_dot.*t5.*t15.*x.*x_dot.*y.*1.22472+beta_dot.*t3.*t20.*x.*x_dot.*y.*1.22472-gamma_dot.*t5.*t14.*x.*y.*y_dot.*7.2646875e-1;
et53 = T_gamma.*t14.*2.970855966714673+T_gamma.*t19.*3.5629477128e-3-t2.*t20.*4.713080655351523e-3-t2.*t22.*7.559910412543251e-3+T_gamma.*t8.*t14.*6.1362+T_gamma.*t8.*t19.*6.00075e-1;
et54 = T_gamma.*t10.*t19.*1.7532+T_beta.*t5.*x.*1.38478628575e+1+T_beta.*t20.*x.*5.0359349556075+beta_dot.*t20.*x_dot.*4.329749032049133e-3+beta_dot.*t22.*x_dot.*1.624091665194202e-3+t2.*t5.*t8.*3.056569529221687e+1;
et55 = t2.*t5.*t14.*(-3.929859463347265)-t2.*t5.*t16.*6.30360217643565-t5.*t6.*t15.*2.260152122742151e-2;
et56 = t5.*t6.*t17.*(-9.792752004982599e-3)-t3.*t6.*t20.*2.710600556380867e-5-t2.*t8.*t20.*1.725481027987207e+1;
et57 = t3.*t6.*t22.*(-1.174444798034242e-5)-t2.*t8.*t22.*1.13017943162159e+1-t2.*t10.*t20.*2.31913956392829+t6.*t11.*t16.*4.289287682949187;
et58 = t2.*t10.*t22.*(-3.770427399426776)+t7.*t11.*t16.*4.289287682949187-t6.*t11.*t18.*4.289287682949187-t2.*t12.*t22.*2.48315625e+1-t2.*t14.*t20.*6.311162086848193;
et59 = t6.*t11.*t19.*8.90219755125e-1+t7.*t11.*t19.*8.90219755125e-1+t6.*t11.*t21.*3.28882818655125e-1+t7.*t11.*t21.*3.84345300655125e-1+t6.*t13.*t21.*(8.1e+1./3.2e+1)-t6.*t15.*t20.*9.804496452962942e-3+t7.*t13.*t21.*(8.1e+1./3.2e+1);
et60 = t2.*t15.*y.*(-6.557421832530962)+t6.*t14.*y.*1.508507113392871+t7.*t14.*y.*1.508507113392871-t6.*t16.*y.*9.599211127015562e-1;
et61 = t7.*t16.*y.*6.425690291983333e-1-t6.*t18.*y.*4.546029721842959e-1+t6.*t19.*y.*1.809152658231802e-3+t7.*t19.*y.*1.809152658231802e-3;
et62 = t6.*t21.*y.*6.579192186818463e-4+t7.*t21.*y.*7.706330695762743e-4+T_beta.*t5.*t14.*x.*5.0359349556075+T_beta.*t10.*t20.*x.*(3.15e+2./8.0)+T_gamma.*t3.*t5.*y.*3.59406e-1+T_beta.*t15.*x.*y.*6.1362;
et63 = beta_dot.*t5.*t14.*x_dot.*3.610230007033025+beta_dot.*t5.*t16.*x_dot.*1.354199613061963+beta_dot.*t8.*t20.*x_dot.*1.24425+beta_dot.*t8.*t22.*x_dot.*4.60827495054675e-1+beta_dot.*t10.*t20.*x_dot.*2.1305156895;
et64 = beta_dot.*t10.*t22.*x_dot.*8.115037575723e-1+beta_dot.*t12.*t22.*x_dot.*(2.43e+2./4.0e+1)+beta_dot.*t14.*t20.*x_dot.*1.355823704727157+beta_dot.*t17.*x_dot.*y.*1.336885185021603-gamma_dot.*t11.*t21.*y_dot.*7.8894e-1+gamma_dot.*t19.*x.*x_dot.*4.74843217383675e-2;
et65 = gamma_dot.*t21.*x.*x_dot.*1.726822096277812e-2-gamma_dot.*t16.*y.*y_dot.*1.336885185021603-gamma_dot.*t21.*y.*y_dot.*1.60332647076e-3+t3.*t5.*t6.*t8.*9.12475249003125e-2-t3.*t5.*t7.*t8.*4.380771414970125e-1;
et66 = t3.*t5.*t6.*t10.*1.82495049800625e-1+t3.*t5.*t7.*t10.*1.82495049800625e-1+t2.*t5.*t8.*t14.*2.998578957015639-t2.*t5.*t8.*t16.*1.301987175023465e+1-t2.*t5.*t10.*t14.*7.932988935e-1;
et67 = t2.*t5.*t10.*t16.*(-4.207791216973153e+1)-t5.*t6.*t8.*t15.*4.515765857389434e-1-t2.*t3.*t11.*t19.*3.8697507-t5.*t7.*t8.*t15.*1.593118023206433e-1-t5.*t6.*t8.*t17.*1.795383920733014e-1;
et68 = t5.*t6.*t10.*t15.*(-1.161286212785119e-1)-t2.*t3.*t11.*t21.*5.0904703125-t3.*t6.*t8.*t20.*1.422271073894344e-2+t5.*t7.*t10.*t15.*7.773623733211313e-2-t3.*t7.*t8.*t20.*1.593118023206433e-1;
et69 = t5.*t6.*t10.*t17.*1.216519821021344+t5.*t6.*t12.*t15.*5.1890625e-1-t3.*t6.*t8.*t22.*1.755752756158312e-2+t3.*t6.*t10.*t20.*5.302852609268813e-2+t5.*t7.*t12.*t15.*5.1890625e-1+t2.*t8.*t10.*t20.*8.691046875e+1;
et70 = t3.*t7.*t10.*t20.*7.773623733211313e-2-t5.*t6.*t12.*t17.*5.1890625e-1-t3.*t6.*t10.*t22.*4.254095911224105e-3+t3.*t6.*t12.*t20.*5.1890625e-1-t2.*t8.*t10.*t22.*8.691046875e+1+t3.*t7.*t12.*t20.*5.1890625e-1+t3.*t6.*t12.*t22.*7.5036375e-1-t2.*t8.*t14.*t20.*2.432166606645056e+1;
et71 = t2.*t10.*t14.*t20.*(-4.584833956915831e+1)+t6.*t8.*t11.*t21.*(8.1e+1./3.2e+1)-t2.*t11.*t15.*t19.*5.0904703125-t2.*t12.*t14.*t20.*2.48315625e+1-t6.*t8.*t15.*t20.*1.970959196348845e-1+t6.*t11.*t14.*t19.*3.727950746479312;
et72 = t6.*t10.*t15.*t20.*1.21226572511012+t7.*t11.*t14.*t19.*4.673632983604313-t6.*t11.*t14.*t21.*1.19595767905125e-1-t6.*t11.*t16.*t19.*4.408883450854312+t6.*t13.*t14.*t19.*(8.1e+1./3.2e+1)+t6.*t12.*t15.*t20.*2.314575e-1+t7.*t13.*t14.*t19.*(8.1e+1./3.2e+1)-t6.*t13.*t14.*t21.*(8.1e+1./3.2e+1);
et73 = t6.*t13.*t16.*t19.*(-8.1e+1./3.2e+1)+t3.*t4.*t5.*x.*4.725869682156708e+1+t4.*t5.*t15.*x.*1.71861698609537e+1+t3.*t4.*t20.*x.*1.71861698609537e+1+t4.*t11.*t21.*x.*2.48315625e+1;
et74 = t2.*t3.*t19.*y.*(-4.832879269443772e-1)-t2.*t3.*t21.*y.*7.625924882280298e-1+t6.*t8.*t14.*y.*3.1157691429375+t7.*t8.*t14.*y.*3.1157691429375-t6.*t8.*t16.*y.*1.942250602925813;
et75 = t7.*t8.*t16.*y.*1.133085365011688-t6.*t8.*t18.*y.*1.133085365011688+t6.*t8.*t19.*y.*8.90219755125e-1+t6.*t8.*t21.*y.*3.23738675717625e-1-t2.*t15.*t19.*y.*7.625924882280298e-1+t7.*t8.*t21.*y.*1.8983372625e-2;
et76 = t6.*t14.*t19.*y.*5.447004972537325e-1+t7.*t14.*t19.*y.*6.433396622679096e-1-t6.*t14.*t21.*y.*1.729905624728822e-3;
et77 = t6.*t16.*t19.*y.*(-4.563328778090248e-1)+t4.*t16.*x.*y.*2.094105194574786e+1+t4.*t19.*x.*y.*8.73305579777625+t4.*t21.*x.*y.*3.175876408789901+T_beta.*t5.*t10.*t14.*x.*(3.15e+2./8.0)+T_gamma.*t3.*t5.*t8.*y.*(3.15e+2./8.0);
et78 = beta_dot.*gamma_dot.*t3.*t19.*x.*3.018681604826212+beta_dot.*gamma_dot.*t3.*t21.*x.*1.097778362627294-beta_dot.*gamma_dot.*t10.*t17.*x.*8.086635e-2+beta_dot.*gamma_dot.*t11.*t22.*x.*6.15346875e-1;
et79 = beta_dot.*gamma_dot.*t15.*t19.*x.*1.097778362627294+T_beta.*t3.*t19.*x.*y.*6.1362+beta_dot.*gamma_dot.*t20.*x.*y.*2.164124224708875e-1+beta_dot.*gamma_dot.*t22.*x.*y.*7.870087206695464e-2+beta_dot.*t5.*t8.*t14.*x_dot.*1.225266627375;
et80 = beta_dot.*t5.*t8.*t16.*x_dot.*5.30881620804675e-1+beta_dot.*t5.*t10.*t16.*x_dot.*1.045602313907805e+1+beta_dot.*t3.*t11.*t21.*x_dot.*2.034315+beta_dot.*t8.*t10.*t22.*x_dot.*(5.67e+2./1.6e+2)+beta_dot.*t8.*t14.*t20.*x_dot.*9.9170911585935e-1+beta_dot.*t10.*t14.*t20.*x_dot.*1.126752689665035e+1+beta_dot.*t11.*t15.*t19.*x_dot.*2.034315;
et81 = beta_dot.*t12.*t14.*t20.*x_dot.*(2.43e+2./4.0e+1)-beta_dot.*t3.*t19.*x.*y_dot.*4.3763203161945e-2+beta_dot.*t3.*t19.*x_dot.*y.*4.367557163475e-1-beta_dot.*t3.*t21.*x.*y_dot.*1.591499329827845e-2+beta_dot.*t3.*t21.*x_dot.*y.*1.654306784478315e-1-beta_dot.*t11.*t22.*x.*y_dot.*(8.1e+1./3.2e+1);
et82 = beta_dot.*t15.*t19.*x.*y_dot.*(-1.591499329827845e-2)+beta_dot.*t15.*t19.*x_dot.*y.*1.502315863469434+gamma_dot.*t3.*t5.*t8.*y_dot.*6.231538285875+gamma_dot.*t5.*t8.*t15.*y_dot.*2.266170730023375-gamma_dot.*t5.*t10.*t15.*y_dot.*1.617327e-1;
et83 = gamma_dot.*t3.*t8.*t20.*y_dot.*2.266170730023375-gamma_dot.*t3.*t10.*t20.*y_dot.*1.617327e-1-gamma_dot.*t11.*t14.*t19.*y_dot.*7.8894e-1+gamma_dot.*t10.*t21.*x.*x_dot.*1.35016875e-1+gamma_dot.*t14.*t19.*x.*x_dot.*1.726822096277812e-2-beta_dot.*t20.*x.*y.*y_dot.*8.90219755125e-1-beta_dot.*t22.*x.*y.*y_dot.*3.23738675717625e-1;
et84 = gamma_dot.*t8.*t21.*y.*y_dot.*(-2.7003375e-1)-gamma_dot.*t14.*t19.*y.*y_dot.*1.338488511492363+t5.*t6.*t8.*t10.*t15.*5.1890625e-1-t5.*t7.*t8.*t10.*t15.*1.35016875e-1+t5.*t6.*t8.*t10.*t17.*1.35016875e-1+t3.*t6.*t8.*t10.*t20.*5.1890625e-1-t3.*t7.*t8.*t10.*t20.*1.35016875e-1+t3.*t6.*t8.*t10.*t22.*1.35016875e-1-t2.*t8.*t10.*t14.*t20.*8.691046875e+1;
et85 = t6.*t8.*t11.*t14.*t19.*(8.1e+1./3.2e+1)+t6.*t8.*t10.*t15.*t20.*2.7003375e-1+t4.*t5.*t10.*t15.*x.*1.382450840274375e+2+t3.*t4.*t10.*t20.*x.*1.382450840274375e+2+t4.*t11.*t14.*t19.*x.*2.48315625e+1+t2.*t3.*t8.*t19.*y.*1.562693219836875e+2-t2.*t3.*t8.*t21.*y.*2.44392238125e+1-t2.*t8.*t15.*t19.*y.*2.44392238125e+1;
et86 = t6.*t8.*t14.*t19.*y.*(-4.729136927208188)+t7.*t8.*t14.*t19.*y.*1.152068737636687-t6.*t8.*t14.*t21.*y.*2.285154102648375-t6.*t8.*t16.*t19.*y.*3.418239467660063+t4.*t14.*t19.*x.*y.*2.411692835453776e+1;
et87 = beta_dot.*gamma_dot.*t5.*t14.*x.*y.*(-1.82495049800625e-1)+beta_dot.*gamma_dot.*t5.*t16.*x.*y.*1.27125759723161+beta_dot.*gamma_dot.*t14.*t20.*x.*y.*1.349958469298564+beta_dot.*t8.*t10.*t14.*t20.*x_dot.*(5.67e+2./1.6e+2)-beta_dot.*t3.*t8.*t19.*x_dot.*y.*1.35016875e-1+beta_dot.*t3.*t8.*t21.*x_dot.*y.*9.965025e-1-beta_dot.*t3.*t10.*t21.*x.*y_dot.*5.1890625e-1;
et88 = beta_dot.*t8.*t15.*t19.*x_dot.*y.*9.965025e-1-beta_dot.*t10.*t15.*t19.*x.*y_dot.*5.1890625e-1-beta_dot.*t11.*t14.*t20.*x.*y_dot.*(8.1e+1./3.2e+1)+gamma_dot.*t10.*t14.*t19.*x.*x_dot.*1.35016875e-1-beta_dot.*t5.*t16.*x.*y.*y_dot.*1.93921452e-2-beta_dot.*t14.*t20.*x.*y.*y_dot.*3.43130820917625e-1-gamma_dot.*t8.*t14.*t19.*y.*y_dot.*2.7003375e-1+gamma_dot.*t5.*t15.*x.*x_dot.*y.*2.10410298e-2;
et89 = gamma_dot.*t3.*t20.*x.*x_dot.*y.*2.10410298e-2-beta_dot.*gamma_dot.*t3.*t10.*t19.*x.*1.78043951025-beta_dot.*gamma_dot.*t5.*t11.*t16.*x.*1.30784625+beta_dot.*gamma_dot.*t3.*t10.*t21.*x.*8.031734692588125-beta_dot.*gamma_dot.*t3.*t12.*t21.*x.*(8.1e+1./1.6e+1)+beta_dot.*gamma_dot.*t10.*t15.*t19.*x.*7.950868342588125-beta_dot.*gamma_dot.*t11.*t14.*t20.*x.*6.92499375e-1-beta_dot.*gamma_dot.*t12.*t15.*t19.*x.*(8.1e+1./1.6e+1);
et90 = T_gamma.*t14.*2.66889011383505e+1+T_gamma.*t19.*3.20080005e-2+t2.*t20.*1.163291677980999e-1-t2.*t22.*7.095244335692625e-3+T_gamma.*t8.*t14.*(4.41e+2./8.0)+T_gamma.*t8.*t19.*(6.3e+1./4.0)+T_gamma.*t10.*t19.*(6.3e+1./4.0)+T_beta.*t5.*x.*6.00075e-1-T_beta.*t20.*x.*2.21445;
et91 = beta_dot.*t20.*x_dot.*7.83967383675e-5-beta_dot.*t22.*x_dot.*2.89306598805e-4+t2.*t5.*t8.*1.32451554375+t2.*t5.*t14.*9.6997550936369e+1-t2.*t5.*t16.*5.916154451064253;
et92 = t5.*t6.*t15.*(-2.099232344482776)-t5.*t6.*t17.*8.148044578175612e-1-t3.*t6.*t20.*2.51760945808553e-3+t2.*t8.*t20.*5.1407523724725e+1;
et93 = t3.*t6.*t22.*(-9.771950279268265e-4)+t2.*t10.*t20.*5.7241451018475e+1-t2.*t10.*t22.*3.4913176875-t2.*t14.*t20.*5.923249695399946+t6.*t11.*t19.*3.857625e-2+t7.*t11.*t19.*3.857625e-2-t6.*t11.*t21.*1.423575e-1;
et94 = t7.*t11.*t21.*3.5589375e-1-t6.*t15.*t20.*8.15781652845488e-1-t2.*t15.*y.*5.890907703762414e+1+t6.*t14.*y.*6.536874428814562e-2+t7.*t14.*y.*6.536874428814562e-2;
et95 = t6.*t16.*y.*(-3.065982835772079e-1)+t7.*t16.*y.*6.030738482226558e-1+t6.*t18.*y.*1.08553292680078+t6.*t19.*y.*7.83967383675e-5+t7.*t19.*y.*7.83967383675e-5;
et96 = t6.*t21.*y.*(-2.89306598805e-4)+t7.*t21.*y.*7.232664970125e-4-T_beta.*t5.*t14.*x.*2.21445+T_gamma.*t3.*t5.*y.*3.22875+T_beta.*t15.*x.*y.*(4.41e+2./8.0)+beta_dot.*t5.*t14.*x_dot.*6.536874428814562e-2-beta_dot.*t5.*t16.*x_dot.*2.412295392890623e-1;
et97 = beta_dot.*t10.*t20.*x_dot.*3.857625e-2-beta_dot.*t10.*t22.*x_dot.*1.423575e-1-beta_dot.*t14.*t20.*x_dot.*2.415188458878673e-1+beta_dot.*t17.*x_dot.*y.*1.201000551225773e+1-gamma_dot.*t11.*t21.*y_dot.*(5.67e+2./8.0e+1)+gamma_dot.*t19.*x.*x_dot.*2.057657175e-3-gamma_dot.*t21.*x.*x_dot.*7.59334905e-3;
et98 = gamma_dot.*t16.*y.*y_dot.*(-1.201000551225773e+1)-gamma_dot.*t21.*y.*y_dot.*1.4403600225e-2+t3.*t5.*t6.*t8.*3.954065625e-3-t3.*t5.*t7.*t8.*1.8983372625e-2+t3.*t5.*t6.*t10.*7.90813125e-3+t3.*t5.*t7.*t10.*7.90813125e-3+t2.*t5.*t8.*t14.*1.954572338021625e+2;
et99 = t2.*t5.*t8.*t16.*(-1.221961190625e+1)-t2.*t5.*t10.*t14.*7.1266584375-t5.*t6.*t8.*t15.*4.36946664375-t2.*t3.*t11.*t19.*3.47641875e+1+t5.*t7.*t8.*t15.*7.005412575e-2-t5.*t6.*t8.*t17.*1.612896232691362-t5.*t6.*t10.*t15.*3.709141875e-2;
et100 = t3.*t6.*t8.*t20.*(-1.25884164375)+t5.*t7.*t10.*t15.*7.295821875e-2+t3.*t7.*t8.*t20.*7.005412575e-2+t5.*t6.*t10.*t17.*6.136327549878862-t3.*t6.*t8.*t22.*4.60827495054675e-1-t3.*t6.*t10.*t20.*1.26800946675+t3.*t7.*t10.*t20.*7.295821875e-2;
et101 = t3.*t6.*t10.*t22.*(-4.73641159442175e-1)+t3.*t6.*t12.*t22.*(5.67e+2./1.6e+2)-t2.*t8.*t14.*t20.*1.221961190625e+1-t2.*t10.*t14.*t20.*3.4913176875-t6.*t8.*t15.*t20.*2.073723727746038-t6.*t11.*t14.*t19.*1.8093375e-1+t6.*t10.*t15.*t20.*5.662686390436688;
et102 = t7.*t11.*t14.*t19.*3.5589375e-1+t6.*t11.*t14.*t21.*1.3670775+t6.*t11.*t16.*t19.*1.3670775+t6.*t12.*t15.*t20.*(5.67e+2./1.6e+2)+t3.*t4.*t5.*x.*2.047880079910148-t4.*t5.*t15.*x.*7.557268746335085-t3.*t4.*t20.*x.*7.557268746335085;
et103 = t2.*t3.*t19.*y.*1.166384779968375e+1-t2.*t3.*t21.*y.*7.157201259375e-1+t6.*t8.*t14.*y.*1.35016875e-1+t7.*t8.*t14.*y.*1.35016875e-1-t6.*t8.*t16.*y.*2.7003375e-1-t7.*t8.*t16.*y.*4.9825125e-1+t6.*t8.*t18.*y.*4.9825125e-1+t6.*t8.*t19.*y.*3.857625e-2-t6.*t8.*t21.*y.*1.423575e-1;
et104 = t2.*t15.*t19.*y.*(-7.157201259375e-1)+t7.*t8.*t21.*y.*4.9825125e-1-t6.*t14.*t19.*y.*4.955566093724848e-1+t7.*t14.*t19.*y.*6.037971147196683e-1-t6.*t14.*t21.*y.*9.727092701408588e-2;
et105 = t6.*t16.*t19.*y.*9.882619997866945e-1+t4.*t16.*x.*y.*1.881254666584125e+2+t4.*t19.*x.*y.*3.784330125e-1-t4.*t21.*x.*y.*1.396527075+beta_dot.*gamma_dot.*t3.*t19.*x.*1.308097417382362e-1;
et106 = beta_dot.*gamma_dot.*t3.*t21.*x.*(-4.827257136061946e-1)-beta_dot.*gamma_dot.*t10.*t17.*x.*7.2646875e-1-beta_dot.*gamma_dot.*t15.*t19.*x.*4.827257136061946e-1+T_beta.*t3.*t19.*x.*y.*(4.41e+2./8.0)+beta_dot.*gamma_dot.*t20.*x.*y.*9.377886375e-3-beta_dot.*gamma_dot.*t22.*x.*y.*3.460710825e-2-beta_dot.*t5.*t8.*t14.*x_dot.*1.35016875e-1;
et107 = beta_dot.*t5.*t8.*t16.*x_dot.*4.9825125e-1+beta_dot.*t5.*t10.*t16.*x_dot.*1.4529375+beta_dot.*t3.*t11.*t21.*x_dot.*(5.67e+2./8.0e+1)+beta_dot.*t8.*t14.*t20.*x_dot.*4.9825125e-1+beta_dot.*t10.*t14.*t20.*x_dot.*1.31058+beta_dot.*t11.*t15.*t19.*x_dot.*(5.67e+2./8.0e+1)-beta_dot.*t3.*t19.*x.*y_dot.*1.89640845e-3+beta_dot.*t3.*t19.*x_dot.*y.*7.90813125e-3+beta_dot.*t3.*t21.*x.*y_dot.*6.9982947e-3;
et108 = beta_dot.*t3.*t21.*x_dot.*y.*(-1.4779687275e-2)+beta_dot.*t15.*t19.*x.*y_dot.*6.9982947e-3+beta_dot.*t15.*t19.*x_dot.*y.*1.199522582498273e+1+gamma_dot.*t3.*t5.*t8.*y_dot.*2.7003375e-1-gamma_dot.*t5.*t8.*t15.*y_dot.*9.965025e-1-gamma_dot.*t5.*t10.*t15.*y_dot.*1.4529375-gamma_dot.*t3.*t8.*t20.*y_dot.*9.965025e-1-gamma_dot.*t3.*t10.*t20.*y_dot.*1.4529375;
et109 = gamma_dot.*t11.*t14.*t19.*y_dot.*(-5.67e+2./8.0e+1)-gamma_dot.*t14.*t19.*x.*x_dot.*7.59334905e-3-beta_dot.*t20.*x.*y.*y_dot.*3.857625e-2+beta_dot.*t22.*x.*y.*y_dot.*1.423575e-1-gamma_dot.*t8.*t21.*y.*y_dot.*(5.67e+2./8.0e+1)-gamma_dot.*t14.*t19.*y.*y_dot.*1.202440911248273e+1-t5.*t7.*t8.*t10.*t15.*(5.67e+2./1.6e+2)+t5.*t6.*t8.*t10.*t17.*(5.67e+2./1.6e+2)-t3.*t7.*t8.*t10.*t20.*(5.67e+2./1.6e+2)+t3.*t6.*t8.*t10.*t22.*(5.67e+2./1.6e+2);
et110 = t6.*t8.*t10.*t15.*t20.*(5.67e+2./8.0e+1)+t4.*t5.*t10.*t15.*x.*3.47641875e+1+t3.*t4.*t10.*t20.*x.*3.47641875e+1+t2.*t3.*t8.*t19.*y.*8.691046875e+1-t2.*t3.*t8.*t21.*y.*8.691046875e+1-t2.*t8.*t15.*t19.*y.*8.691046875e+1-t6.*t8.*t14.*t19.*y.*4.1239125e-1+t6.*t8.*t14.*t21.*y.*4.9825125e-1+t6.*t8.*t16.*t19.*y.*9.965025e-1;
et111 = t4.*t14.*t19.*x.*y.*1.867289395834125e+2-beta_dot.*gamma_dot.*t5.*t14.*x.*y.*7.90813125e-3+beta_dot.*gamma_dot.*t5.*t16.*x.*y.*1.204582622933272e+1+beta_dot.*gamma_dot.*t14.*t20.*x.*y.*1.201121912108272e+1+beta_dot.*t3.*t8.*t21.*x_dot.*y.*(5.67e+2./1.6e+2)-beta_dot.*t3.*t10.*t21.*x.*y_dot.*(5.67e+2./1.6e+2)+beta_dot.*t8.*t15.*t19.*x_dot.*y.*(5.67e+2./1.6e+2)-beta_dot.*t10.*t15.*t19.*x.*y_dot.*(5.67e+2./1.6e+2);
et112 = beta_dot.*t5.*t16.*x.*y.*y_dot.*(-1.7421075e-1)-beta_dot.*t14.*t20.*x.*y.*y_dot.*3.185325e-2-gamma_dot.*t8.*t14.*t19.*y.*y_dot.*(5.67e+2./8.0e+1)+gamma_dot.*t5.*t15.*x.*x_dot.*y.*1.89023625e-1+gamma_dot.*t3.*t20.*x.*x_dot.*y.*1.89023625e-1-beta_dot.*gamma_dot.*t3.*t10.*t19.*x.*7.71525e-2-beta_dot.*gamma_dot.*t5.*t11.*t16.*x.*(5.67e+2./8.0e+1)+beta_dot.*gamma_dot.*t3.*t10.*t21.*x.*1.146200625+beta_dot.*gamma_dot.*t10.*t15.*t19.*x.*4.19731875e-1;
et113 = beta_dot.*gamma_dot.*t11.*t14.*t20.*x.*(-5.67e+2./8.0e+1);
out1 = [x_dot;t51.*(et1+et2+et3+et4+et5+et6+et7+et8+et9+et10+et11+et12+et13+et14+et15+et16+et17+et18+et19+et20+et21+et22+et23+et24+et25+et26+et27+et28+et29+et30+et31+et32+et33+et34+et35+et36);beta_dot;-t51.*(et37+et38+et39+et40+et41+et42+et43+et44+et45+et46+et47+et48+et49+et50+et51+et52);y_dot;t51.*(et53+et54+et55+et56+et57+et58+et59+et60+et61+et62+et63+et64+et65+et66+et67+et68+et69+et70+et71+et72+et73+et74+et75+et76+et77+et78+et79+et80+et81+et82+et83+et84+et85+et86+et87+et88+et89);gamma_dot;t51.*(et90+et91+et92+et93+et94+et95+et96+et97+et98+et99+et100+et101+et102+et103+et104+et105+et106+et107+et108+et109+et110+et111+et112+et113)];

== matlab function Repetitive_Controller/Chart/Init/x_Setpoint_Function ==
  data: t input; x_setpoint_symfun output
function x_setpoint_symfun = x_setpoint(t)
%#codegen

%    This function was generated by the Symbolic Math Toolbox version 9.0.
%    10-Dec-2021 15:41:40

t2 = t./3.0;
t3 = t.*pi.*(2.0./3.0);
t4 = -t2;
t6 = sin(t3);
t5 = exp(t4);
t7 = t5-1.0;
x_setpoint_symfun = [t6.*t7.*(-3.0./2.0e+1);(t5.*t6)./2.0e+1-(t7.*pi.*cos(t3))./1.0e+1];

== stateflow chart Repetitive_Controller/Chart ==
  state Init
  state time_fun [function]
  state Run
  (default) -> Init
  Init -> Run : [t>3*T]{Run.x = Init.x, t_f = t}
  Run -> Run : [(t-t_f)>= T]{time_fun, tf = t}
  data: sf_internal_action_state_placeholder_data local double size=1 =0; x local; sf_internal_action_state_placeholder_data local double size=1 =0; x local; T parameter; input output; state output; t_f data_store_memory

== matlab function Repetitive_Controller/Chart/Init/y_Setpoint_Function ==
  data: t input; y_setpoint_symfun output
function y_setpoint_symfun = y_setpoint(t)
%#codegen

%    This function was generated by the Symbolic Math Toolbox version 9.0.
%    10-Dec-2021 15:41:40

t2 = t./3.0;
t3 = t.*pi.*(2.0./3.0);
t4 = -t2;
t6 = cos(t3);
t7 = sin(t3);
t5 = exp(t4);
t8 = t5-1.0;
y_setpoint_symfun = [t6.*t7.*t8.*(-3.0./2.0e+1);(t5.*t6.*t7)./2.0e+1-(t6.^2.*t8.*pi)./1.0e+1+(t7.^2.*t8.*pi)./1.0e+1];
